simulink model "ProposedProblem4"  (R2013a)
settings: Solver=ode45  StartTime=0.0  StopTime=2629746  RelTol=1e-3
undefined symbols (not defined in the file): des, gcbh
settings Model: Creator=gabig  LastModifiedBy=gabig

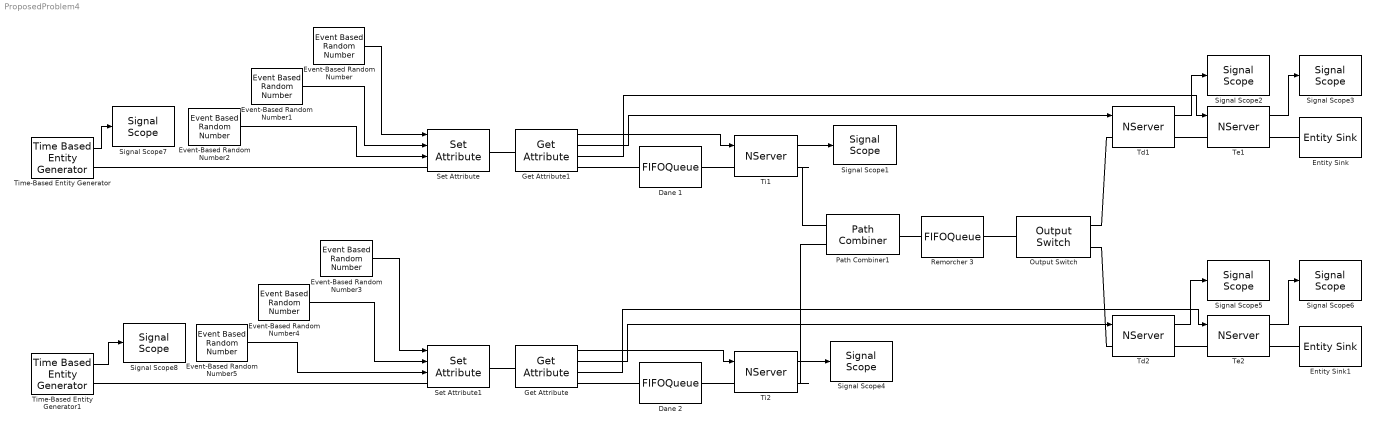
== system ProposedProblem4 ==
  Dane 1 : FIFOQueue
  Dane 2 : FIFOQueue
  Entity Sink : EntitySink
  Entity Sink1 : EntitySink
  Event-Based Random Number : EventBasedRandomNumber  Distribution=Uniform  minUnif=780  maxUnif=1620  Seed=12145
  Event-Based Random Number1 : EventBasedRandomNumber  Distribution=Uniform  minUnif=36000  maxUnif=50400  Seed=12245
  Event-Based Random Number2 : EventBasedRandomNumber  Distribution=Uniform  minUnif=1200  maxUnif=1800  Seed=12445
  Event-Based Random Number3 : EventBasedRandomNumber  Distribution=Uniform  minUnif=1980  maxUnif=3420  Seed=12545
  Event-Based Random Number4 : EventBasedRandomNumber  Distribution=Uniform  minUnif=57600  maxUnif=86400  Seed=12365
  Event-Based Random Number5 : EventBasedRandomNumber  Distribution=Uniform  minUnif=1500  maxUnif=2100  Seed=12645
  Get Attribute : GetAttribute  AttributeName=Ti|Td|Te  AttributeMissing=Error|Error|Error  AttributeDefaultValue=1|1|1  AttributeTreatAsVector=1|1|1  AttributeSendTiming=After entity departure|After entity departure|After entity departure  EvaluatedDefaultAttributeValue={ [];[];[]}
      settings: OutputPortMap=o1,o2,o3
  Get Attribute1 : GetAttribute  AttributeName=Ti|Td|Te  AttributeMissing=Error|Error|Error  AttributeDefaultValue=1|1|1  AttributeTreatAsVector=1|1|1  AttributeSendTiming=After entity departure|After entity departure|After entity departure  EvaluatedDefaultAttributeValue={ [];[];[]}
      settings: OutputPortMap=o1,o2,o3
  Output Switch : OutputSwitch  NumberOutputPorts=2
  Path Combiner1 : PathCombiner  NumberInputPorts=2
  Remorcher 3 : FIFOQueue
  Set Attribute : SetAttribute  AttributeName=Attribute1|Ti|Td|Te  AttributeFrom=Dialog|Signal port|Signal port|Signal port  AttributeValue=1|1|1|1  AttributeTreatAsVector=1|1|1|1  EvaluatedAttributeValue={ 1;[];[];[]}
      settings: InputPortMap=u1,u2,u3
  Set Attribute1 : SetAttribute  AttributeName=Attribute1|Ti|Td|Te  AttributeFrom=Dialog|Signal port|Signal port|Signal port  AttributeValue=2|1|1|1  AttributeTreatAsVector=1|1|1|1  EvaluatedAttributeValue={ 2;[];[];[]}
      settings: InputPortMap=u1,u2,u3
  Signal Scope{1..8} (8 alike) : SignalScope  LoadFcn=des.scope.CallbackSupport('seLoadFcn',gcbh)  StartFcn=des.scope.CallbackSupport('seStartFcn',gcbh)  StopFcn=des.scope.CallbackSupport('seStopFcn',gcbh)
      settings: CopyFcn=des.scope.CallbackSupport('seCopyFcn',gcbh)  DeleteFcn=des.scope.CallbackSupport('seDeleteFcn',gcbh)  PreSaveFcn=des.scope.CallbackSupport('sePreSaveFcn',gcbh)  NameChangeFcn=des.scope.CallbackSupport('seNameChangeFcn',gcbh)  OpenFcn=des.scope.CallbackSupport('seOpenFcn',gcbh)
  Td1 : NServer  ServiceTimeFrom=Signal port t  StatAverageWait=on
      settings: OutputPortMap=o4
  Td2 : NServer  ServiceTimeFrom=Signal port t  StatAverageWait=on
      settings: OutputPortMap=o4
  Te1 : NServer  ServiceTimeFrom=Signal port t  StatAverageWait=on
      settings: OutputPortMap=o4
  Te2 : NServer  ServiceTimeFrom=Signal port t  StatAverageWait=on
      settings: OutputPortMap=o4
  Ti1 : NServer  NumberOfServers=6  ServiceTimeFrom=Signal port t  StatAverageWait=on
      settings: OutputPortMap=o4
  Ti2 : NServer  NumberOfServers=3  ServiceTimeFrom=Signal port t  StatAverageWait=on
      settings: OutputPortMap=o4
  Time-Based Entity Generator : TimeBasedEntityGenerator  Distribution=Uniform  Minimum=6000  Maximum=9600  StatNumberDeparted=on
  Time-Based Entity Generator1 : TimeBasedEntityGenerator  Distribution=Uniform  InitialSeed=12399  Minimum=11580  Maximum=12420  StatNumberDeparted=on
  wires:
  Event-Based Random Number/1 -> Set Attribute/1
  Event-Based Random Number1/1 -> Set Attribute/2
  Event-Based Random Number2/1 -> Set Attribute/3
  Event-Based Random Number3/1 -> Set Attribute1/1
  Event-Based Random Number4/1 -> Set Attribute1/2
  Event-Based Random Number5/1 -> Set Attribute1/3
  Get Attribute1/2 -> Td1/1
  Get Attribute1/3 -> Te1/1
  Get Attribute/1 -> Ti2/1
  Get Attribute/2 -> Td2/1
  Time-Based Entity Generator/1 -> Signal Scope7/1
  Ti1/1 -> Signal Scope1/1
  Td1/1 -> Signal Scope2/1
  Te1/1 -> Signal Scope3/1
  Td2/1 -> Signal Scope5/1
  Ti2/1 -> Signal Scope4/1
  Te2/1 -> Signal Scope6/1
  Time-Based Entity Generator1/1 -> Signal Scope8/1
  Get Attribute1/1 -> Ti1/1
  Get Attribute/3 -> Te2/1
  connections:
  Set Attribute1/RConn1 -- Get Attribute/LConn1
  Ti1/RConn1 -- Path Combiner1/LConn1
  Dane 2/RConn1 -- Ti2/LConn1
  Dane 1/RConn1 -- Ti1/LConn1
  Time-Based Entity Generator/RConn1 -- Set Attribute/LConn1
  Ti2/RConn1 -- Path Combiner1/LConn2
  Time-Based Entity Generator1/RConn1 -- Set Attribute1/LConn1
  Get Attribute1/RConn1 -- Dane 1/LConn1
  Te1/RConn1 -- Entity Sink/LConn1
  Get Attribute/RConn1 -- Dane 2/LConn1
  Path Combiner1/RConn1 -- Remorcher 3/LConn1
  Set Attribute/RConn1 -- Get Attribute1/LConn1
  Remorcher 3/RConn1 -- Output Switch/LConn1
  Output Switch/RConn1 -- Td1/LConn1
  Td1/RConn1 -- Te1/LConn1
  Td2/RConn1 -- Te2/LConn1
  Te2/RConn1 -- Entity Sink1/LConn1
  Output Switch/RConn2 -- Td2/LConn1
